simulink model "exampleMaxRunTime"  (R2016b)
settings: Solver=ode45  StartTime=0.0  StopTime=30  MaxStep=5  RelTol=1e-3  EnableMultiTasking=on
libraries: carnot x3
settings Model: Creator=drhf  LastModifiedBy=drhf
settings DataIOCC: LimitDataPoints=on  SaveFormat=Array  SignalLoggingSaveFormat=ModelDataLogs
settings OptimizationCC: ExpressionDepthLimit=2147483647  LifeSpan=inf
settings DebuggingCC: SolverPrmCheckMsg=warning  StateNameClashWarn=warning  SFUnexpectedBacktrackingDiag=warning  SFNoUnconditionalDefaultTransitionDiag=warning  SFExecutionAtInitializationDiag=none
settings HardwareCC: ProdBitPerPointer=32  ProdBitPerSizeT=32  ProdBitPerPtrDiffT=32  ProdLargestAtomicFloat=None  ProdIntDivRoundTo=Undefined  ProdEndianess=Unspecified  ProdWordSize=32  ProdHWDeviceType=32-bit Generic
settings ModelReferenceCC: PropagateSignalLabelsOutOfModel=off
settings GRTTargetCC: TargetLangStandard=C89/C90 (ANSI)  GeneratePreprocessorConditionals=Disable all  CombineOutputUpdateFcns=off  GRTInterface=on
settings ConfigComp: CovMetricSettings=dw  CovHtmlReporting=on  CovSaveCumulativeToWorkspaceVar=on  CovSaveSingleToWorkspaceVar=on  CovExternalEMLEnable=off

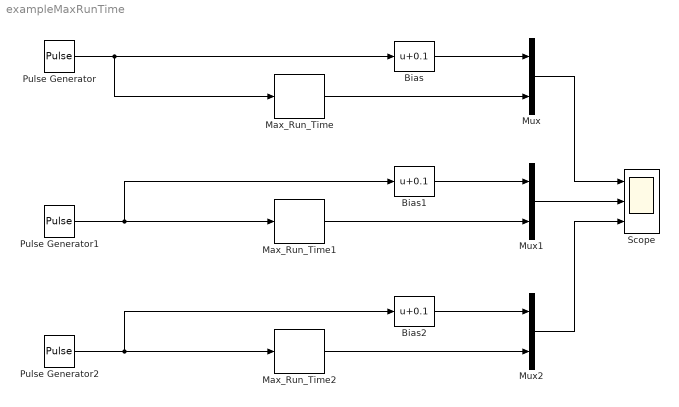
== system exampleMaxRunTime ==
  Bias : Bias  Bias=0.1
  Bias1 : Bias  Bias=0.1
  Bias2 : Bias  Bias=0.1
  Max_Run_Time : carnot/Control/Max_Run_Time  tmaxrun=5
  Max_Run_Time1 : carnot/Control/Max_Run_Time  tmaxrun=5
  Max_Run_Time2 : carnot/Control/Max_Run_Time  tmaxrun=5
  Mux : Mux  Inputs=2
  Mux1 : Mux  Inputs=2
  Mux2 : Mux  Inputs=2
  Pulse Generator : DiscretePulseGenerator  PulseType=Time based  Amplitude=2  Period=10  PulseWidth=80
  Pulse Generator1 : DiscretePulseGenerator  PulseType=Time based  Amplitude=2  Period=10  PulseWidth=10
  Pulse Generator2 : DiscretePulseGenerator  PulseType=Time based  Amplitude=2  Period=20  PulseWidth=90
  Scope : Scope  NumInputPorts=3
  wires:
  Pulse Generator/1 -> Max_Run_Time/1, Bias/1
  Mux/1 -> Scope/1
  Max_Run_Time/1 -> Mux/2
  Pulse Generator1/1 -> Max_Run_Time1/1, Bias1/1
  Max_Run_Time1/1 -> Mux1/2
  Mux1/1 -> Scope/2
  Bias/1 -> Mux/1
  Bias1/1 -> Mux1/1
  Pulse Generator2/1 -> Bias2/1, Max_Run_Time2/1
  Max_Run_Time2/1 -> Mux2/2
  Mux2/1 -> Scope/3
  Bias2/1 -> Mux2/1
